simulink model "sm_excv_trackI2R4_1_float"  (R2026a)
settings: Solver=ode23t  StopTime=20  FixedStep=2e-4  AbsTol=1e-3
StartFcn:
  | tic
StopFcn:
  | Elapsed_Sim_Time = toc;
  | disp(['Elapsed Sim Time = ' num2str(Elapsed_Sim_Time)]);
undefined symbols (not defined in the file or in its folder): Excv
libraries: sm_lib x3, fl_lib x2, nesl_utility x2, sm_excv_chassis_lib x1, sm_trackV_lib_chain_underc_elem x1, simulink x1, sm_trackV_lib_chain_lower_frame_s46i2u0l4 x1
CloseFcn:
  | try,close(h1_sm_excv_track_single_float),end
  | clear h1_sm_excv_track_single_float
  | try,close(h2_sm_excv_track_single_float),end
  | clear h2_sm_excv_track_single_float
  | try,close(h3_sm_excv_track_single_float),end
  | clear h3_sm_excv_track_single_float
  | try,close(h4_sm_excv_track_single_float),end
  | clear h4_sm_excv_track_single_float
  | 
  | 
  | clear simlog_sm_excv_track_single_float
  | clear logsout_sm_excv_track_single_float
Description:
  | Excavator Track (Single, Two Idler) Suspended in Air
  | Copyright 2023-2026 The MathWorks, Inc.
settings Model: Creator=evo  LastModifiedBy=smiller
settings SolverCC: ExtrapolationOrder=1.0
settings DataIOCC: SignalLoggingName=logsout_sm_excv_trackI2R4_1_float
settings DebuggingCC: SymbolicDimsDataTypeCodeGenerationDiagnostic=none
settings SimscapeCC: SimscapeNominalValues="[{\"value\":\"1\",\"unit\":\"A\"},{\"value\":\"1\",\"unit\":\"bar\"},{\"value\":\"1\",\"unit\":\"cm^2\"},{\"value\":\"1\",\"unit\":\"cm^3/s\"},{\"value\":\"1\",\"unit\":\"kJ/kg\"},{\"value\":\"1\",\"unit\":\"kW\"},{\"value\":\"1\",\"unit\":\"l\"},{\"value\":\"1\",\"unit\":\"N\"},{\"value\":\"1\",\"unit\":\"N*m\"},{\"value\":\"1\",\"unit\":\"V\"}]"  SimscapeLogSimulationStatistics=on  SimscapeLogName=simlog_sm_excv_trackI2R4_1_float  SimscapeLogLimitData=off
settings DiagnosticsConfigSet: SimMechanicsConflictingReferenceFrames=none
settings ExplorerConfigSet: InternalSimMechanicsExplorerSettings="<ExplorerConfiguration><canonicalview>default</canonicalview><AnimationSetting><BasePlaybackSpeed>1.0</BasePlaybackSpeed><PlaybackSpeedFactor>1.0</PlaybackSpeedFactor></AnimationSetting><TilePanel><TileInfo><Tiles Columns=\"1\" Count=\"1\" Rows=\"1\"><Column Weight=\"1\"/><Row Weight=\"1\"/><Tile Height=\"1\" Width=\"1\" X=\"0\" Y=\"0\"/></Tiles></TileInfo><SceneInfo><SceneViewer><BGColor><R>1</R><G>1</G><B>1</B></BGColor><Camera><DoPerspective>off</DoPerspective><Position><X>1.0619723079055905</X><Y>0.0999999850762665066</Y><Z>0.10502998201713698</Z></Position><Center><X>1.0619723079055905</X><Y>1.09999998507626651</Y><Z>0.10502998201713698</Z></Center><Up><X>0</X><Y>-0</Y><Z>1</Z></Up><ViewLimDist>1</ViewLimDist><YLim>0.433967051489734801</YLim><XLim>0.698744305372238195</XLim></Camera></SceneViewer></SceneInfo></TilePanel><MechEditorPanel><Cameras/><GfxPanelCameraMap/><VideoCreator><PlaybackSpeedRatio>1.0</PlaybackSpeedRatio><FrameRate>30</FrameRate><VideoFormat>Motion JPEG AVI</VideoFormat><FrameSize>auto</FrameSize></VideoCreator></MechEditorPanel></ExplorerConfiguration>"

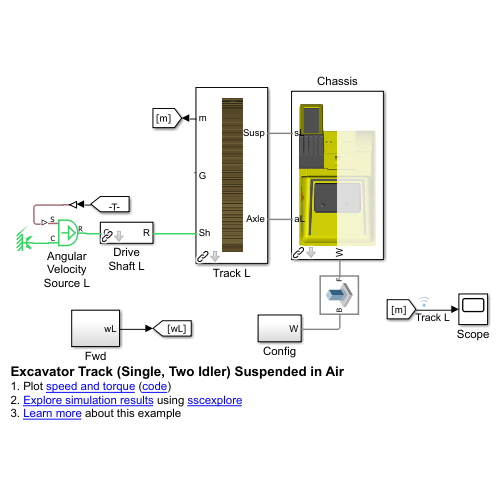
[thumbnail: Simulink's stored preview of the top-level diagram]
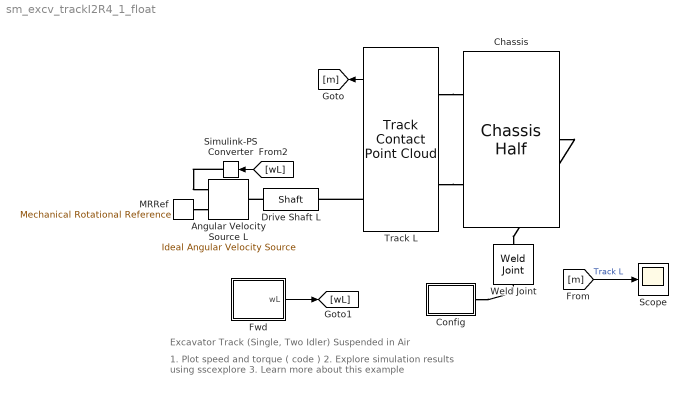
== system sm_excv_trackI2R4_1_float ==
  note: Excavator Track (Single, Two Idler) Suspended in Air
  note: 1. Plot speed and torque ( code )
      | 2. Explore simulation results using sscexplore
      | 3. Learn more about this example
  Angular Velocity Source L : fl_lib/Mechanical/Mechanical Sources/Ideal Angular Velocity Source
  Chassis : sm_excv_chassis_lib/Chassis Half  Camera=Excv.Chassis.Camera  offset_cg=Excv.Chassis.CGOffset  offset_axle=Excv.Chassis.AxleOffset  offset_sprk2axle_x=Excv.Frame.AxleX  offset_sprk2axle_y=Excv.Frame.AxleY  track_sep_ctr=Excv.Chassis.TrackSepCtr  chassis_mass=Excv.Chassis.Mass/2  chassis_moi=Excv.Chassis.MOI/2  chassis_poi=Excv.Chassis.POI/2
  Config : Subsystem
  Drive Shaft L : sm_trackV_lib_chain_underc_elem/Shaft  k_shaft=Excv.Drive.Shaft.k  b_shaft=Excv.Drive.Shaft.b
  Fwd : Subsystem  VariantControl=Fwd
  MRRef : fl_lib/Mechanical/Rotational Elements/Mechanical Rotational Reference
  Scope : Scope
      settings: ActiveDisplayYMinimum=-11747.25975  ActiveDisplayYMaximum=35828.2276
  Simulink-PS Converter : nesl_utility/Simulink-PS Converter  PhysicalDomain=network_engine_domain  SubClassName=ps_input  LeftPortType=input  RightPortType=output  PseudoPeriodic=off  Frequencies=[]  NoiseDistribution=none  NoiseParameters=[]  Unit=1  AffineConversion=off  FilteringAndDerivatives=provide  SimscapeFilterOrder=1  InputFilterTimeConstant=0.001  UdotUserProvided=0
  Track L : sm_trackV_lib_chain_lower_frame_s46i2u0l4/Track Contact Point Cloud  popup_leftOrRight=Left  sprk_xc=ExcvI2R4.Sprocket.sprocket_xc  sprk_len=ExcvI2R4.Sprocket.sprk_width  sprk_rho=ExcvI2R4.Sprocket.density  sprk_clr=ExcvI2R4.Sprocket.clr  sprk_opc=ExcvI2R4.Sprocket.opc  sprk_contact_geo_ptcld=ExcvI2R4.Sprocket.teeth_contact.ptcld.pts  sprk_contact_geo_rad=ExcvI2R4.Sprocket.teeth_contact.ptcld.rad  sprk_contact_geo_clr=ExcvI2R4.Sprocket.teeth_contact.ptcld.clr  sprk_contact_geo_opc=ExcvI2R4.Sprocket.teeth_contact.ptcld.opc  idlerR_rad=ExcvI2R4.IdlerR.rad  idlerF_rad=ExcvI2R4.IdlerF.rad  idlerR_len=ExcvI2R4.IdlerR.len  idlerF_len=ExcvI2R4.IdlerF.len  idlerR_rho=ExcvI2R4.IdlerR.rho  idlerF_rho=ExcvI2R4.IdlerF.rho  idlerR_clr=ExcvI2R4.IdlerR.clr  idlerF_clr=ExcvI2R4.IdlerF.clr  idlerR_opc=ExcvI2R4.IdlerR.opc  idlerF_opc=ExcvI2R4.IdlerF.opc  idlerR_contgeo_clr=ExcvI2R4.IdlerR.chain_contact.clr  idlerF_contgeo_clr=ExcvI2R4.IdlerF.chain_contact.clr  idlerR_contgeo_opc=ExcvI2R4.IdlerR.chain_contact.opc  idlerF_contgeo_opc=ExcvI2R4.IdlerF.chain_contact.opc  roller_lower_rad=ExcvI2R4.Roller.Lower.rad  roller_lower_len=ExcvI2R4.Roller.Lower.len  roller_lower_rho=ExcvI2R4.Roller.Lower.rho  roller_lower_clr=ExcvI2R4.Roller.Lower.clr  roller_lower_opc=ExcvI2R4.Roller.Lower.opc  roller_lower_contgeo_clr=[1.0 0.0 0.0]  roller_lower_contgeo_opc=1  tensioner_cyl_len=ExcvI2R4.IdlerF.Tensioner.cyl.len  tensioner_cyl_rad=ExcvI2R4.IdlerF.Tensioner.cyl.rad  tensioner_cyl_rho=ExcvI2R4.IdlerF.Tensioner.cyl.rho  tensioner_cyl_clr=ExcvI2R4.IdlerF.Tensioner.cyl.clr  tensioner_cyl_opc=ExcvI2R4.IdlerF.Tensioner.cyl.opc  tensioner_pist_len=ExcvI2R4.IdlerF.Tensioner.piston.len  tensioner_pist_rad=ExcvI2R4.IdlerF.Tensioner.piston.rad  tensioner_pist_rho=ExcvI2R4.IdlerF.Tensioner.piston.rho  tensioner_pist_clr=ExcvI2R4.IdlerF.Tensioner.piston.clr  tensioner_pist_opc=ExcvI2R4.IdlerF.Tensioner.piston.opc  tensioner_br_len=ExcvI2R4.IdlerF.Tensioner.bracket.len  tensioner_br_width=ExcvI2R4.IdlerF.Tensioner.bracket.wid  tensioner_br_height=ExcvI2R4.IdlerF.Tensioner.bracket.height  tensioner_br_thk=ExcvI2R4.IdlerF.Tensioner.bracket.thk  tensioner_br_rho=ExcvI2R4.IdlerF.Tensioner.bracket.rho  tensioner_br_clr=ExcvI2R4.IdlerF.Tensioner.bracket.clr  tensioner_br_opc=ExcvI2R4.IdlerF.Tensioner.bracket.opc  tensioner_eqpos=ExcvI2R4.IdlerF.Tensioner.xeq  tensioner_x0=ExcvI2R4.IdlerF.Tensioner.x0  tensioner_k=ExcvI2R4.IdlerF.Tensioner.K  tensioner_b=ExcvI2R4.IdlerF.Tensioner.B  roller_lower_x=ExcvI2R4.Frame.Sprk2LowerX  idlerF_x=ExcvI2R4.Frame.IdlerAssyX  idlerR_x=ExcvI2R4.Frame.Sprk2IdlerRX  axle_x=ExcvI2R4.Frame.AxleX  roller_lower_y=ExcvI2R4.Frame.Sprk2LowerY  sprk_pitch_rad=ExcvI2R4.Sprocket.sprocket_rPitch  idlerF_y=ExcvI2R4.Frame.Sprk2IdlerFY  idlerR_y=ExcvI2R4.Frame.Sprk2IdlerFY  axle_y=ExcvI2R4.Frame.AxleY  frame_cg_offset=ExcvI2R4.Frame.CGOffset  frame_mass=ExcvI2R4.Frame.Mass  frame_moi=ExcvI2R4.Frame.MOI  frame_poi=ExcvI2R4.Frame.POI  frame_susp_offset=ExcvI2R4.Frame.SuspOffset  chain_wid=ExcvI2R4.Chain.chain_wid  chain_seg_m=ExcvI2R4.Chain.link_m  chain_seg_cg=ExcvI2R4.Chain.link_cg  chain_seg_moi=ExcvI2R4.Chain.link_moi  chain_seg_poi=ExcvI2R4.Chain.link_poi  plate_xc=ExcvI2R4.Chain.plate_xc  plate_h=ExcvI2R4.Chain.plate_h  pin_sep=ExcvI2R4.Chain.pin_sep  plate_thk=ExcvI2R4.Chain.plate_thk  plate_ang=ExcvI2R4.Chain.plate_ang  plate_clr=ExcvI2R4.Chain.plate_clr  plate_opc=ExcvI2R4.Chain.plate_opc  pin_len=ExcvI2R4.Chain.pin_len  pin_rad=ExcvI2R4.Chain.pin_rad  pin_clr=ExcvI2R4.Chain.pin_clr  pin_opc=ExcvI2R4.Chain.pin_opc  shoe_xc=ExcvI2R4.Shoe.xc  shoe_w=ExcvI2R4.Shoe.w  shoe_m=ExcvI2R4.Shoe.mass  shoe_cg=ExcvI2R4.Shoe.cg  shoe_moi=ExcvI2R4.Shoe.moi  shoe_poi=ExcvI2R4.Shoe.poi  shoe_clr=ExcvI2R4.Shoe.clr  shoe_opc=ExcvI2R4.Shoe.opc  jointTargets=track_joint_targetsC46I2  chainDamping=ExcvI2R4.Chain.damping  ptcld_shoe=ExcvI2R4.Shoe.ground_contact.ptcld.pts  ptcld_shoe_rad=ExcvI2R4.Shoe.ground_contact.ptcld.rad  ptcld_shoe_clr=ExcvI2R4.Shoe.ground_contact.ptcld.clr  ptcld_shoe_opc=ExcvI2R4.Shoe.ground_contact.ptcld.opc  chain_to_roller_clr=ExcvI2R4.Chain.roller_contact.clr  chain_to_roller_opc=ExcvI2R4.Chain.roller_contact.opc  chain_to_teeth_clr=ExcvI2R4.Chain.teeth_contact.clr  chain_to_teeth_opc=ExcvI2R4.Chain.teeth_contact.opc  B_Sprocket=ExcvI2R4.Contact.Sprocket.B  K_Sprocket=ExcvI2R4.Contact.Sprocket.K  TW_Sprocket=ExcvI2R4.Contact.Sprocket.TW  K_Roller=ExcvI2R4.Contact.Roller.K  B_Roller=ExcvI2R4.Contact.Roller.B  TW_Roller=ExcvI2R4.Contact.Roller.TW  K_IdlerF=ExcvI2R4.Contact.IdlerF.K  B_IdlerF=ExcvI2R4.Contact.IdlerF.B  TW_IdlerF=ExcvI2R4.Contact.IdlerF.TW  K_IdlerR=ExcvI2R4.Contact.IdlerR.K  B_IdlerR=ExcvI2R4.Contact.IdlerR.B  TW_IdlerR=ExcvI2R4.Contact.IdlerR.TW  popup_sense_roller=Actuator Torque
  Weld Joint : sm_lib/Joints/Weld Joint  JointMode=Normal  CompositeWrenchDir=FollowerOnBase  CompositeWrenchFrame=BaseFrame  SenseConstraintForce=off  SenseConstraintTorque=off  SenseTotalForce=off  SenseTotalTorque=off
  wires:
  Track L/1 -> [m]
  [m] -> Scope/1  "Track L"
  [wL] -> Simulink-PS Converter/1
  Fwd/1(wL) -> [wL]
  connections:
  Config/LConn1 -- Weld Joint/LConn1
  Chassis/RConn1 -- Weld Joint/RConn1
  Simulink-PS Converter/RConn1 -- Angular Velocity Source L/RConn1
  MRRef/LConn1 -- Angular Velocity Source L/RConn2
  Drive Shaft L/LConn1 -- Angular Velocity Source L/LConn1
  Track L/LConn1 -- Chassis/LConn1
  Track L/LConn2 -- Chassis/LConn2
  Track L/RConn2 -- Drive Shaft L/RConn1

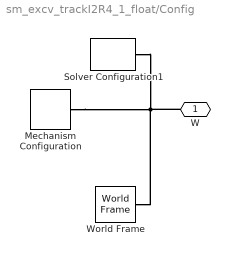
== system sm_excv_trackI2R4_1_float/Config ==
  Mechanism Configuration : sm_lib/Utilities/Mechanism Configuration  UniformGravity=Constant  GravityVector=[-9.80665 0 0]  GravityVectorUnits=m/s^2  LinearizationDelta=0.001  JointModeTransitionNonlinearIterations=2
      settings: AttributesFormatString=Gravity: %<GravityVector>
  Solver Configuration1 : nesl_utility/Solver Configuration  PhysicalDomain=network_engine_domain  SubClassName=solver  LeftPortType=input  RightPortType=generic  Tones=[]  Harmonics=[]  SimulateNoise=off  Profile=off  UseLocalSampling=off  EnableSwitchedLinearOptims=on  FrequencyDomain=off  UseCCode=off  RelTol=0.001  AbsTol=0.001  MinStep=1e-09  ToWorkspace=off  RevertToSquareIcSolve=off  NumHomotopyIterations=100  PhasorMode=off  PhasorModeNumHarmonics=1  ConsistencySolver=NEWTON_FTOL  CanonicalOrdering=UNORDERED  OptimizeIntermediates=UNOPTIMIZED  IndexReductionMethod=DerivativeReplacement  DoDC=off  ResidualTolerance=1e-09  ConsistencyTolSource=GLOBAL  ConsistencyAbsTol=0.001  ConsistencyRelTol=0.001  ConsistencyTolFactor=0.001  UseLocalSolver=off  LocalSolverChoice=NE_BACKWARD_EULER_ADVANCER  ResolveIndetEquations=on  FunctionEvalNumThread=1  LocalSolverSampleTime=0.001  DoFixedCost=off  MaxNonlinIter=3  MaxModeIter=2  ComputeImpulses=off  ImpulseIterations=2  LinearAlgebra=auto  LinearAlgebraNumThread=0  EquationFormulation=NE_TIME_EF  DelaysMemoryBudget=1024  AutomaticFiltering=on  FilteringTimeConstant=0.001  PartitionStorageMethod=AS_NEEDED  PartitionMemoryBudget=1024  PartitionMethod=ROBUST  MultibodyUseLocalSolver=off  MultibodyLocalSolverChoice=ODE1  MultibodyLocalSolverSampleTime=0.001
  World Frame : sm_lib/Frames and Transforms/World Frame
  W : PMIOPort  Side=Left
  connections:
  W/RConn1 -- Solver Configuration1/RConn1 -- Mechanism Configuration/RConn1 -- World Frame/RConn1

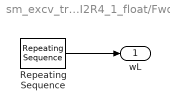
== system sm_excv_trackI2R4_1_float/Fwd ==
  Repeating Sequence : simulink/Sources/Repeating Sequence  rep_seq_t=[0 2 2.01 40]  rep_seq_y=[0 0 3 3]
  wL : Outport
  wires:
  Repeating Sequence/1 -> wL/1
